simulink model "MySimulink"  (R2024a)
settings: Solver=ode45  StartTime=ti  StopTime=tf  FixedStep=dt  MaxStep=1e-3  RelTol=1e-4  AbsTol=1e-6
values from neighbouring files (symbols this model uses):
  index_value = [1 2]    [Start.m]
settings Model: Creator=perruquetti  LastModifiedBy=perruquetti
settings SolverCC: AlgebraicLoopSolver=LineSearch
settings DebuggingCC: AlgebraicLoopMsg=none  UnconnectedInputMsg=warning  UnconnectedOutputMsg=warning  UnconnectedLineMsg=warning
settings ModelReferenceCC: EnableRefExpFcnMdlSchedulingChecks=on
settings RTWCC: GPUComputeCapability=3.5  DLArmComputeVersion=19.05

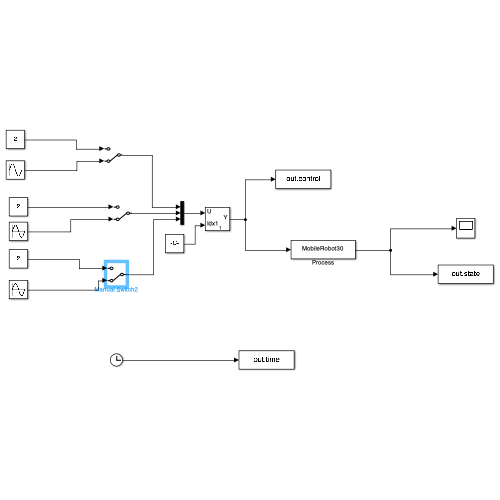
[thumbnail: Simulink's stored preview of the top-level diagram]
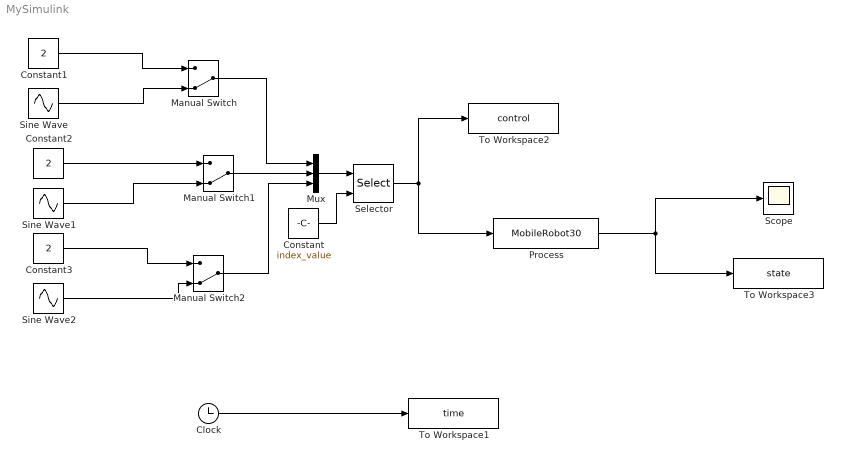
== system MySimulink ==
  Clock : Clock
  Constant : Constant  Value=index_value
  Constant1 : Constant  Value=2
  Constant2 : Constant  Value=2
  Constant3 : Constant  Value=2
  Manual Switch : ManualSwitch  CurrentSetting=0
  Manual Switch1 : ManualSwitch  CurrentSetting=0
  Manual Switch2 : ManualSwitch  CurrentSetting=0
  Mux : Mux  Inputs=3
  Process : S-Function  FunctionName=MobileRobot30  Parameters=Params  SFunctionDeploymentMode=off  EnableBusSupport=off
  Scope : Scope
  Selector : Selector  InputPortWidth=3  IndexOptions=Index vector (port)  Indices=[1]  OutputSizes=1
  Sine Wave : Sin  SampleTime=0
  Sine Wave1 : Sin  SampleTime=0
  Sine Wave2 : Sin  SampleTime=0
  To Workspace1 : ToWorkspace  VariableName=time  SampleTime=-1
  To Workspace2 : ToWorkspace  VariableName=control  SampleTime=-1
  To Workspace3 : ToWorkspace  VariableName=state  SampleTime=-1
  wires:
  Clock/1 -> To Workspace1/1
  Process/1 -> Scope/1, To Workspace3/1
  Constant1/1 -> Manual Switch/1
  Sine Wave/1 -> Manual Switch/2
  Selector/1 -> To Workspace2/1, Process/1
  Mux/1 -> Selector/1
  Manual Switch/1 -> Mux/1
  Constant2/1 -> Manual Switch1/1
  Sine Wave1/1 -> Manual Switch1/2
  Constant3/1 -> Manual Switch2/1
  Sine Wave2/1 -> Manual Switch2/2
  Manual Switch1/1 -> Mux/2
  Manual Switch2/1 -> Mux/3
  Constant/1 -> Selector/2
